simulink model "partFourLinearizedUnicycle"  (R2021b)
settings: Solver=VariableStepAuto  StartTime=0.0  StopTime=10.0  RelTol=1e-3
settings Model: Creator=ericp  LastModifiedBy=ericp

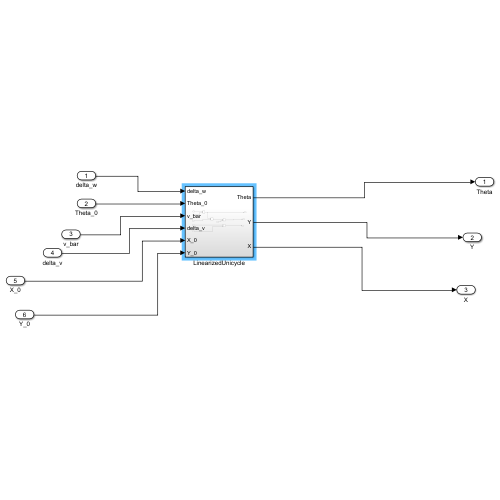
[thumbnail: Simulink's stored preview of the top-level diagram]
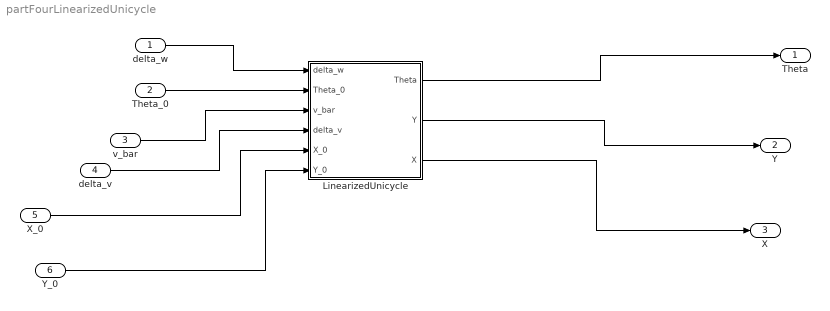
== system partFourLinearizedUnicycle ==
  delta_w : Inport
  Theta_0 : Inport  Port=2
  v_bar : Inport  Port=3
  delta_v : Inport  Port=4
  X_0 : Inport  Port=5
  Y_0 : Inport  Port=6
  LinearizedUnicycle : Subsystem
  Theta : Outport
  Y : Outport  Port=2
  X : Outport  Port=3
  wires:
  delta_w/1 -> LinearizedUnicycle/1(delta_w)
  Theta_0/1 -> LinearizedUnicycle/2(Theta_0)
  v_bar/1 -> LinearizedUnicycle/3(v_bar)
  delta_v/1 -> LinearizedUnicycle/4(delta_v)
  X_0/1 -> LinearizedUnicycle/5(X_0)
  Y_0/1 -> LinearizedUnicycle/6(Y_0)
  LinearizedUnicycle/1(Theta) -> Theta/1
  LinearizedUnicycle/2(Y) -> Y/1
  LinearizedUnicycle/3(X) -> X/1

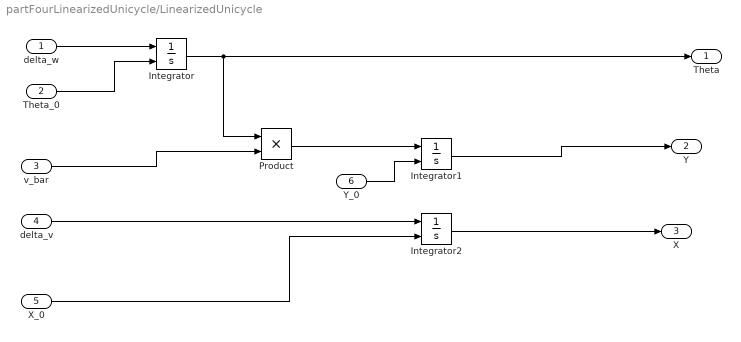
== system partFourLinearizedUnicycle/LinearizedUnicycle ==
  delta_w : Inport
  Theta_0 : Inport  Port=2
  v_bar : Inport  Port=3
  delta_v : Inport  Port=4
  X_0 : Inport  Port=5
  Y_0 : Inport  Port=6
  Integrator : Integrator  InitialConditionSource=external
  Integrator1 : Integrator  InitialConditionSource=external
  Integrator2 : Integrator  InitialConditionSource=external
  Product : Product
  Theta : Outport
  Y : Outport  Port=2
  X : Outport  Port=3
  wires:
  Integrator/1 -> Theta/1, Product/1
  Theta_0/1 -> Integrator/2
  v_bar/1 -> Product/2
  Product/1 -> Integrator1/1
  delta_w/1 -> Integrator/1
  X_0/1 -> Integrator2/2
  Integrator1/1 -> Y/1
  Y_0/1 -> Integrator1/2
  delta_v/1 -> Integrator2/1
  Integrator2/1 -> X/1
